simulink model "Estimator_Tester"  (R2024b)
settings: Solver=FixedStepAuto  StartTime=0.0  StopTime=10  FixedStep=0.001  RelTol=1e-3
values from neighbouring files (symbols this model uses):
  motor_B = 0.0001    [Lab1_motor_params_student.m]
  motor_Eff = 0.5    [Lab1_motor_params_student.m]
  motor_J = 0.001    [Lab1_motor_params_student.m]
  motor_Ke = 0.05    [Lab1_motor_params_student.m]
  motor_L = 0.0038    [Lab1_motor_params_student.m]
  motor_R = 5.54    [Lab1_motor_params_student.m]
libraries: simulink x4, spsStairGeneratorLib x1, eeStairGenerator x1
settings Model: Creator=tanawatp  LastModifiedBy=acer
settings RTWCC: GPUComputeCapability=3.5

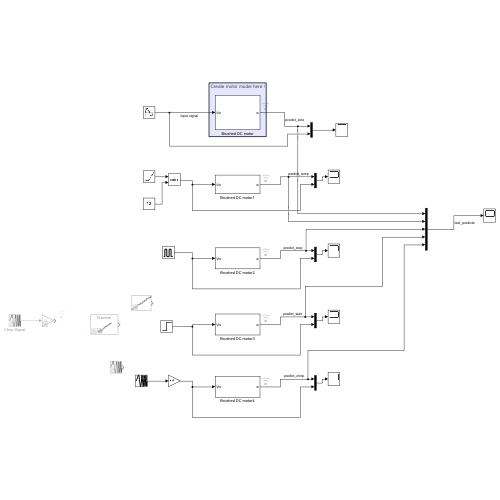
[thumbnail: Simulink's stored preview of the top-level diagram]
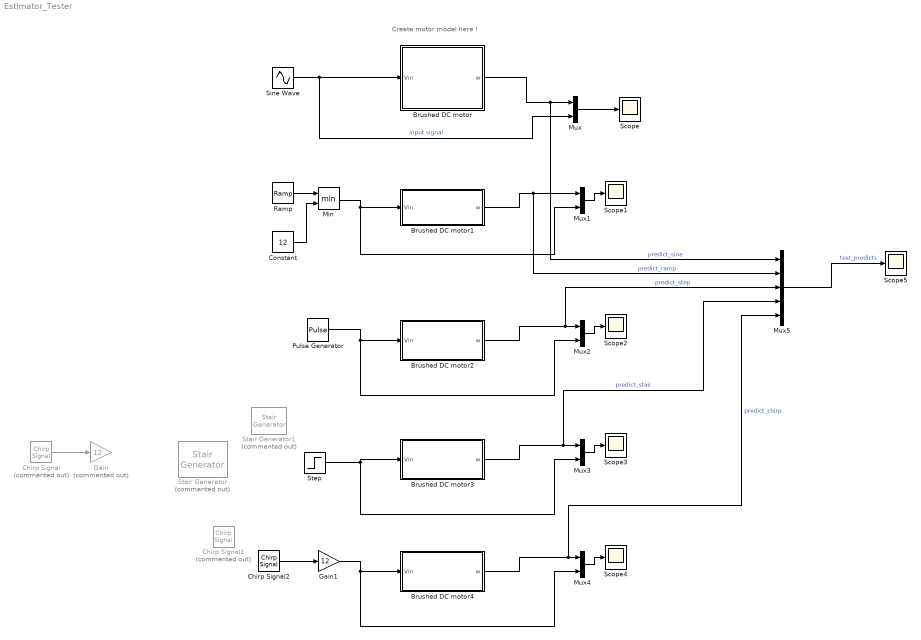
== system Estimator_Tester ==
  note: Create motor model here !
  Brushed DC motor : Subsystem
  Brushed DC motor1 : Subsystem
  Brushed DC motor2 : Subsystem
  Brushed DC motor3 : Subsystem
  Brushed DC motor4 : Subsystem
  Chirp Signal : simulink/Sources/Chirp Signal  Commented=on  f1=0.1  T=40  f2=5
  Chirp Signal1 : simulink/Sources/Chirp Signal  Commented=on  f1=0.05  T=10  f2=20
  Chirp Signal2 : simulink/Sources/Chirp Signal  f1=1  T=10  f2=5
  Constant : Constant  Value=12
  Gain : Gain  Commented=on  Gain=12
  Gain1 : Gain  Gain=12
  Min : MinMax  Inputs=2
  Mux{,1..4} (5 alike) : Mux  Inputs=2
  Mux5 : Mux  Inputs=5
  Pulse Generator : DiscretePulseGenerator  PulseType=Time based  Amplitude=12  Period=1  PulseWidth=50
  Ramp : simulink/Sources/Ramp  slope=12/5  start=0  InitialOutput=0
  Scope{,1..5} (6 alike) : Scope
  Sine Wave : Sin  Amplitude=12  Frequency=2*pi*1  SampleTime=0
  Stair Generator1 : spsStairGeneratorLib/Stair Generator  Commented=on  t=[1 2 3 4 5 6 7 8 9 10]  e=[1.2 2.4 3.6 4.8 6.0 7.2 8.4 9.6 10.8 12.0]  Ts=0
  Stair Generator : eeStairGenerator/Stair Generator  Commented=on  LabelModeActiveChoice=Discrete  TimeInput=[1 2 3 4 5 6 7 8 9 10]  AmplitudeInput=[1.2 2.4 3.6 4.8 6.0 7.2 8.4 9.6 10.8 12.0]  SampleTime=-1  RepeatPattern=off  OutDataTypeStr=double
      settings: LibrarySourceBlock=ee_sl_lib/General Control/Stair Generator
  Step : Step  Time=5  Before=6  After=12  SampleTime=0
  wires:
  Brushed DC motor/1(w) -> Mux5/1, Mux/1  "predict_sine"
  Chirp Signal/1 -> Gain/1
  Sine Wave/1 -> Mux/2, Brushed DC motor/1(Vin)  "input signal"
  Mux/1 -> Scope/1
  Ramp/1 -> Min/1
  Constant/1 -> Min/2
  Min/1 -> Mux1/2, Brushed DC motor1/1(Vin)
  Brushed DC motor1/1(w) -> Mux5/2, Mux1/1  "predict_ramp"
  Mux1/1 -> Scope1/1
  Mux2/1 -> Scope2/1
  Brushed DC motor2/1(w) -> Mux5/3, Mux2/1  "predict_step"
  Pulse Generator/1 -> Mux2/2, Brushed DC motor2/1(Vin)
  Mux3/1 -> Scope3/1
  Brushed DC motor3/1(w) -> Mux5/4, Mux3/1  "predict_stair"
  Step/1 -> Brushed DC motor3/1(Vin), Mux3/2
  Chirp Signal2/1 -> Gain1/1
  Brushed DC motor4/1(w) -> Mux5/5, Mux4/1  "predict_chirp"
  Mux4/1 -> Scope4/1
  Gain1/1 -> Brushed DC motor4/1(Vin), Mux4/2
  Mux5/1 -> Scope5/1  "test_predicts"

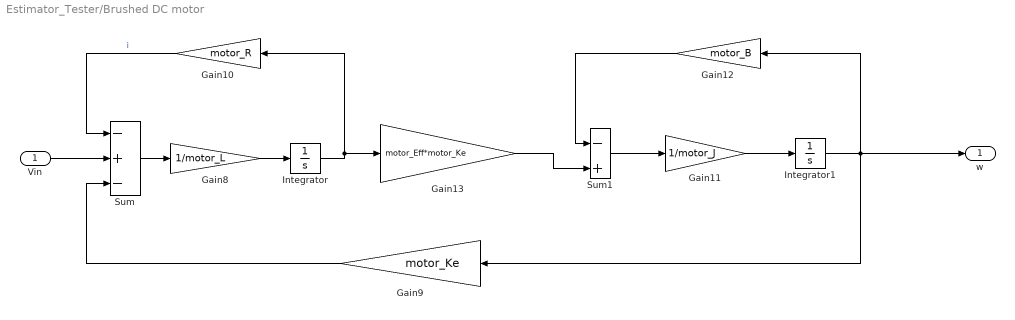
== system Estimator_Tester/Brushed DC motor ==
  Vin : Inport
  Gain10 : Gain  Gain=motor_R
  Gain11 : Gain  Gain=1/motor_J
  Gain12 : Gain  Gain=motor_B
  Gain13 : Gain  Gain=motor_Eff*motor_Ke
  Gain8 : Gain  Gain=1/motor_L
  Gain9 : Gain  Gain=motor_Ke
  Integrator : Integrator
  Integrator1 : Integrator
  Sum : Sum  Inputs=-+-
  Sum1 : Sum  Inputs=-|+|
  w : Outport
  wires:
  Vin/1 -> Sum/2
  Sum/1 -> Gain8/1
  Gain8/1 -> Integrator/1
  Integrator/1 -> Gain10/1, Gain13/1
  Gain10/1 -> Sum/1  "i"
  Gain13/1 -> Sum1/2
  Sum1/1 -> Gain11/1
  Integrator1/1 -> Gain9/1, Gain12/1, w/1
  Gain12/1 -> Sum1/1
  Gain11/1 -> Integrator1/1
  Gain9/1 -> Sum/3

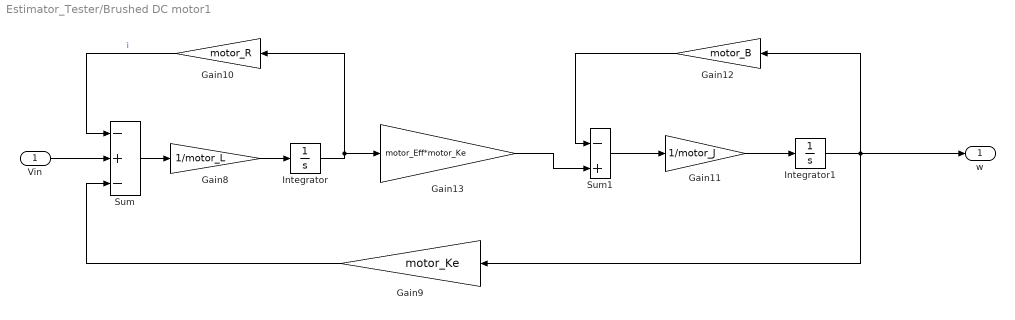
== system Estimator_Tester/Brushed DC motor1 ==
  Vin : Inport
  Gain10 : Gain  Gain=motor_R
  Gain11 : Gain  Gain=1/motor_J
  Gain12 : Gain  Gain=motor_B
  Gain13 : Gain  Gain=motor_Eff*motor_Ke
  Gain8 : Gain  Gain=1/motor_L
  Gain9 : Gain  Gain=motor_Ke
  Integrator : Integrator
  Integrator1 : Integrator
  Sum : Sum  Inputs=-+-
  Sum1 : Sum  Inputs=-|+|
  w : Outport
  wires:
  Gain9/1 -> Sum/3
  Gain11/1 -> Integrator1/1
  Gain12/1 -> Sum1/1
  Integrator1/1 -> w/1, Gain12/1, Gain9/1
  Sum1/1 -> Gain11/1
  Gain13/1 -> Sum1/2
  Gain10/1 -> Sum/1  "i"
  Integrator/1 -> Gain13/1, Gain10/1
  Gain8/1 -> Integrator/1
  Sum/1 -> Gain8/1
  Vin/1 -> Sum/2

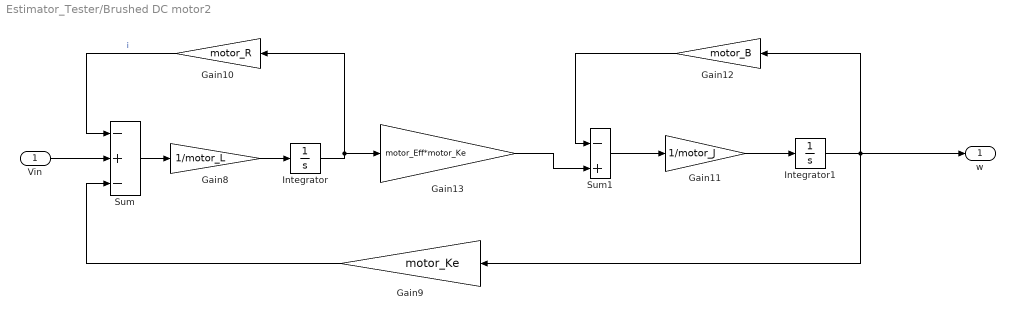
== system Estimator_Tester/Brushed DC motor2 ==
  Vin : Inport
  Gain10 : Gain  Gain=motor_R
  Gain11 : Gain  Gain=1/motor_J
  Gain12 : Gain  Gain=motor_B
  Gain13 : Gain  Gain=motor_Eff*motor_Ke
  Gain8 : Gain  Gain=1/motor_L
  Gain9 : Gain  Gain=motor_Ke
  Integrator : Integrator
  Integrator1 : Integrator
  Sum : Sum  Inputs=-+-
  Sum1 : Sum  Inputs=-|+|
  w : Outport
  wires:
  Gain9/1 -> Sum/3
  Gain11/1 -> Integrator1/1
  Gain12/1 -> Sum1/1
  Integrator1/1 -> w/1, Gain12/1, Gain9/1
  Sum1/1 -> Gain11/1
  Gain13/1 -> Sum1/2
  Gain10/1 -> Sum/1  "i"
  Integrator/1 -> Gain13/1, Gain10/1
  Gain8/1 -> Integrator/1
  Sum/1 -> Gain8/1
  Vin/1 -> Sum/2

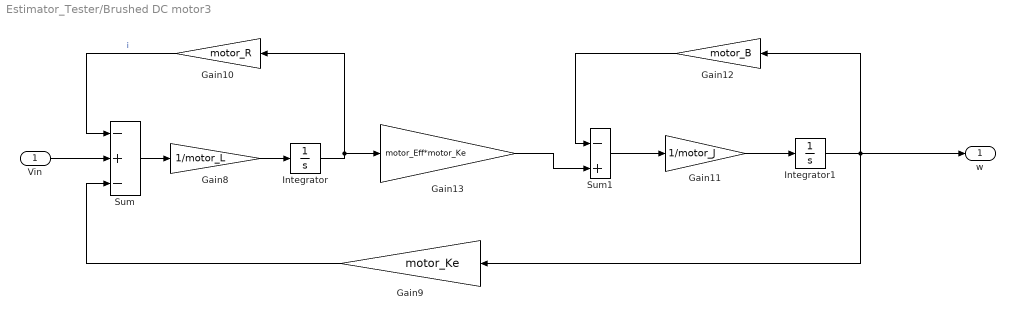
== system Estimator_Tester/Brushed DC motor3 ==
  Vin : Inport
  Gain10 : Gain  Gain=motor_R
  Gain11 : Gain  Gain=1/motor_J
  Gain12 : Gain  Gain=motor_B
  Gain13 : Gain  Gain=motor_Eff*motor_Ke
  Gain8 : Gain  Gain=1/motor_L
  Gain9 : Gain  Gain=motor_Ke
  Integrator : Integrator
  Integrator1 : Integrator
  Sum : Sum  Inputs=-+-
  Sum1 : Sum  Inputs=-|+|
  w : Outport
  wires:
  Gain9/1 -> Sum/3
  Gain11/1 -> Integrator1/1
  Gain12/1 -> Sum1/1
  Integrator1/1 -> w/1, Gain12/1, Gain9/1
  Sum1/1 -> Gain11/1
  Gain13/1 -> Sum1/2
  Gain10/1 -> Sum/1  "i"
  Integrator/1 -> Gain13/1, Gain10/1
  Gain8/1 -> Integrator/1
  Sum/1 -> Gain8/1
  Vin/1 -> Sum/2

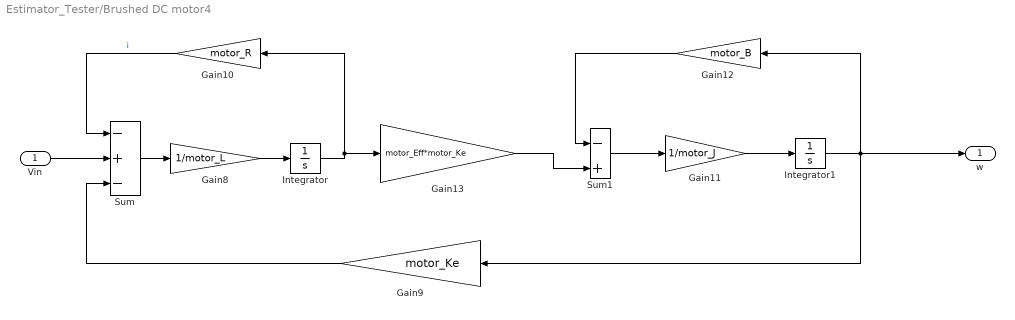
== system Estimator_Tester/Brushed DC motor4 ==
  Vin : Inport
  Gain10 : Gain  Gain=motor_R
  Gain11 : Gain  Gain=1/motor_J
  Gain12 : Gain  Gain=motor_B
  Gain13 : Gain  Gain=motor_Eff*motor_Ke
  Gain8 : Gain  Gain=1/motor_L
  Gain9 : Gain  Gain=motor_Ke
  Integrator : Integrator
  Integrator1 : Integrator
  Sum : Sum  Inputs=-+-
  Sum1 : Sum  Inputs=-|+|
  w : Outport
  wires:
  Vin/1 -> Sum/2
  Sum/1 -> Gain8/1
  Gain8/1 -> Integrator/1
  Integrator/1 -> Gain10/1, Gain13/1
  Gain10/1 -> Sum/1  "i"
  Gain13/1 -> Sum1/2
  Sum1/1 -> Gain11/1
  Integrator1/1 -> Gain9/1, Gain12/1, w/1
  Gain12/1 -> Sum1/1
  Gain11/1 -> Integrator1/1
  Gain9/1 -> Sum/3
